simulink model "AirTableModel"  (R2021a)
settings: Solver=FixedStepAuto  StartTime=0.0  StopTime=endTime  FixedStep=dynamicsRate  RelTol=1e-3  EnableMultiTasking=on
InitFcn:
  | loadThrusterData
  | loadSensorData
values from neighbouring files (symbols this model uses):
  AccelIIR_Den = [1.000000000000000  -1.561018075800718   0.641351538057563]    [loadSensorData.m]
  AccelIIR_Num = [0.020083365564211   0.040166731128423   0.020083365564211]    [loadSensorData.m]
  cameraVec = [1 0 0]    [loadSensorData.m]
  controlRate = 0.025    [loadBusData.m]
  controlType = 1    [loadBusData.m]    (also in loadControlData.m = 2)
  dynamicsRate = 0.005    [loadBusData.m]
  finalRangeAttitude = [0 0 90]*dtr    [loadGuidanceData.m]
  finalRangeValue = 0.25    [loadGuidanceData.m]
  initialCovariance = diag([999999 999999 999999 999999 999999 999999])    [loadSensorData.m]
  initialNavState = [initialState + [0.01 -0.01 1e-3 0 0 1e-3]]    [loadSensorData.m]
  Kd = [x(4) x(5) 0 0 0 x(6)]    [executeSim.m]    (also in loadBusData.m = [500.0000  501.0938 0 0 0 18.4778]; loadControlData.m = [80 80 0 0 0 5] .*[.2 .2  0 0 0 .1]; planarPIDControl.m = [kd(1) 0 0; 0 kd(2) 0; 0 0 kd(3)])
  Ki = [x(7) x(8) 0 0 0 x(9)]    [executeSim.m]    (also in loadBusData.m = [1.0000    1.0313   0 0 0 58.1181]; loadControlData.m = [4  4  0 0 0 1] .*[1   1  0 0 0 .5]; planarPIDControl.m = [ki(1) 0 0; 0 ki(2) 0; 0 0 ki(3)])
  Kp = [x(1) x(2) 0 0 0 x(3)]    [executeSim.m]    (also in loadBusData.m = [500.0000  246.1321 0 0 0 50.1701]; loadControlData.m = [70 70 0 0 0 20].*[.2 .2  0 0 0 .25]; planarPIDControl.m = [kp(1) 0 0; 0 kp(2) 0; 0 0 kp(3)])
  M_Tracker_To_Body = [1 0 0; 0 1 0; 0 0 1]    [loadSensorData.m]
  measurementNoise = [1 .0873 0.0017 2].* [.01 1 1 .01]    [loadSensorData.m]
  processNoise = 0    [loadSensorData.m]
  R_Tracker_To_ECEF = [0 0 0]    [loadSensorData.m]
  rangeSensorAngBody = [0; 90*dtr; 180*dtr; 270*dtr]    [loadSensorData.m]
  rangeSensorFOV = [0*dtr; 0*dtr; 0*dtr; 0*dtr]    [loadSensorData.m]
  rangeSensorIdx = 1    [loadGuidanceData.m]
  SMGains = x    [executeSim.m]    (also in loadBusData.m = [2.0801    3.0489    8.9333    4.9881    3.0029    9.5293   ; loadControlData.m = [3.5078    3.9888    6.3119    1.8214    4.7749    7.3059   )
  useRangeGuid = 0    [loadGuidanceData.m]
  VelIIR_Den = [1.000000000000000  -1.944477657767094   0.945977936232282]    [loadSensorData.m]
  VelIIR_Num = [0.375069616296964   0.750139232593927   0.375069616296964]*1e-3    [loadSensorData.m]
  wallBounds = [wallA; wallB; wallC; wallD]    [loadSensorData.m]
undefined symbols (not defined in the file or in its folder): initialState, navType, PPGains, rangeSensorLocBody, refIdx, targetVec
libraries: simulink x25
(part 2 of 2)

== system AirTableModel/Executive/Guidance/RangeSensorGuidance ==
  In1 : Inport
  rangeSensorData : Inport  Port=2
  Bus Selector2 : BusSelector  OutputSignals=TranState_ECEF.R_Sys_ECEF,RotState_Body_ECEF.ECEF_To_Body_Euler,TranState_ECEF.V_Sys_ECEF,RotState_Body_ECEF.BodyRates_wrt_ECEF_In_Body
  Mux3 : Mux
  RangeGuidance : ModelReference  ModelNameDialog=RangeGuidance  SimulationMode=Normal  ModelReferenceVersion=6.8
      settings: PortSchema="{\"entries\":[{\"content\":{\"sides\":[{\"content\":{\"connectorIds\":[\"In1\",\"In2\",\"In4\",\"In3\",\"In6\",\"In5\"]},\"type\":\"ConnectorPlacement.EquallySpacedRectSide\",\"uuid\":\"ce2fad76-9ac2-4efb-9069-bf35fa3b239d\"},{\"content\":{\"connectorIds\":[\"Out1\",\"Out2\",\"Out3\",\"Out4\",\"Out5\"],\"side\":\"RIGHT\"},\"type\":\"ConnectorPlacement.EquallySpacedRectSide\",\"uuid\":\"aa89394c-f584-49d8-8867-538537a392b4\"},{\"content\":{\"connectorIds\":[],\"side\":\"TOP\"},\"type\":\"ConnectorPlacement.EquallySpacedRectSide\",\"uuid\":\"b335fb80-6985-455b-ae93-e5936637ca43\"}]},\"type\":\"ConnectorPlacement.EquallySpacedConnector\",\"uuid\":\"e071ca64-4f20-42cf-9888-09e4aeb0f4d6\"}],\"packageUris\":[\"http://schema.mathworks.com/mf0/Connector/R2020b\"],\"version\":\"1.0\"}"
  To Workspace4 : ToWorkspace  VariableName=sensorBodyVec1  SaveFormat=Timeseries  SampleTime=-1
  To Workspace5 : ToWorkspace  VariableName=rangeError1  SaveFormat=Timeseries  SampleTime=-1
  To Workspace6 : ToWorkspace  VariableName=rangeErrorECEF1  SaveFormat=Timeseries  SampleTime=-1
  To Workspace7 : ToWorkspace  VariableName=desiredPosECEF1  SaveFormat=Timeseries  SampleTime=-1
  To Workspace8 : ToWorkspace  VariableName=sensorECEFVec1  SaveFormat=Timeseries  SampleTime=-1
  rangeAttitude : Constant  Value=finalRangeAttitude
  rangeSensorAngle : Constant  Value=rangeSensorAngBody
  rangeSensorIdx : Constant  Value=rangeSensorIdx
  rangeValue : Constant  Value=finalRangeValue
  desiredPosECEF : Outport
  wires:
  In1/1 -> Bus Selector2/1
  Bus Selector2/3 -> Mux3/3  "<V_Sys_ECEF>"
  RangeGuidance/3 -> To Workspace5/1
  Mux3/1 -> RangeGuidance/1
  rangeAttitude/1 -> RangeGuidance/2
  Bus Selector2/4 -> Mux3/4  "<BodyRates_wrt_ECEF_In_Body>"
  Bus Selector2/2 -> Mux3/2  "<ECEF_To_Body_Euler>"
  RangeGuidance/2 -> To Workspace4/1
  rangeSensorData/1 -> RangeGuidance/4
  RangeGuidance/4 -> To Workspace6/1
  Bus Selector2/1 -> Mux3/1  "<R_Sys_ECEF>"
  RangeGuidance/1 -> desiredPosECEF/1, To Workspace7/1
  RangeGuidance/5 -> To Workspace8/1
  rangeSensorIdx/1 -> RangeGuidance/3
  rangeSensorAngle/1 -> RangeGuidance/5
  rangeValue/1 -> RangeGuidance/6

== system AirTableModel/Executive/Guidance/ReferenceTrajectoryGuidance ==
  Time : Inport
  refTraj : Inport  Port=2
  controlType : Inport  Port=3
  If : If  IfExpression=u1 == 3
  LookupRefTrajInterpolate : Subsystem  TreatAsAtomicUnit=on
  LookupRefTrajNoInterp : Subsystem  TreatAsAtomicUnit=on
  Merge : Merge
  referenceValues : Outport
  wires:
  refTraj/1 -> LookupRefTrajInterpolate/2(refTraj), LookupRefTrajNoInterp/2(refTraj)
  Merge/1 -> referenceValues/1
  controlType/1 -> If/1
  If/1 -> LookupRefTrajNoInterp/Action
  If/2 -> LookupRefTrajInterpolate/Action
  LookupRefTrajNoInterp/1(referenceValues) -> Merge/1
  LookupRefTrajInterpolate/1(referenceValues) -> Merge/2
  Time/1 -> LookupRefTrajInterpolate/1(Time), LookupRefTrajNoInterp/1(Time)

== system AirTableModel/Navigation/FilterSensorData/FilterVector ==
  Signal : Inport
  Numerator : Inport  Port=2
  Denominator : Inport  Port=3
  IC : Inport  Port=4
  Discrete Filter : DiscreteFilter  NumeratorSource=Input port  DenominatorSource=Input port  InitialStatesSource=Input port  a0EqualsOne=on
      settings: InputPortMap=u0,p1,p3,p5
  Discrete Filter1 : DiscreteFilter  NumeratorSource=Input port  DenominatorSource=Input port  InitialStatesSource=Input port  a0EqualsOne=on
      settings: InputPortMap=u0,p1,p3,p5
  Discrete Filter2 : DiscreteFilter  NumeratorSource=Input port  DenominatorSource=Input port  InitialStatesSource=Input port  a0EqualsOne=on
      settings: InputPortMap=u0,p1,p3,p5
  Mux1 : Mux  Inputs=3
  X : Selector  InputPortWidth=3  IndexOptions=Index vector (dialog)  Indices=1  OutputSizes=1
  X3 : Selector  InputPortWidth=3  IndexOptions=Index vector (dialog)  Indices=1  OutputSizes=1
  Y : Selector  InputPortWidth=3  IndexOptions=Index vector (dialog)  Indices=2  OutputSizes=1
  Y3 : Selector  InputPortWidth=3  IndexOptions=Index vector (dialog)  Indices=2  OutputSizes=1
  Z : Selector  InputPortWidth=3  IndexOptions=Index vector (dialog)  Indices=3  OutputSizes=1
  Z3 : Selector  InputPortWidth=3  IndexOptions=Index vector (dialog)  Indices=3  OutputSizes=1
  Out1 : Outport
  wires:
  Signal/1 -> Z/1, Y/1, X/1
  IC/1 -> Z3/1, X3/1, Y3/1
  Mux1/1 -> Out1/1
  Discrete Filter/1 -> Mux1/1
  X/1 -> Discrete Filter/1
  X3/1 -> Discrete Filter/4
  Y/1 -> Discrete Filter1/1
  Y3/1 -> Discrete Filter1/4
  Z/1 -> Discrete Filter2/1
  Z3/1 -> Discrete Filter2/4
  Discrete Filter1/1 -> Mux1/2
  Discrete Filter2/1 -> Mux1/3
  Numerator/1 -> Discrete Filter1/2, Discrete Filter/2, Discrete Filter2/2
  Denominator/1 -> Discrete Filter2/3, Discrete Filter1/3, Discrete Filter/3

== system AirTableModel/Navigation/FilterSensorData/FilterVector1 ==
  Signal : Inport
  Numerator : Inport  Port=2
  Denominator : Inport  Port=3
  IC : Inport  Port=4
  Discrete Filter : DiscreteFilter  NumeratorSource=Input port  DenominatorSource=Input port  InitialStatesSource=Input port  a0EqualsOne=on
      settings: InputPortMap=u0,p1,p3,p5
  Discrete Filter1 : DiscreteFilter  NumeratorSource=Input port  DenominatorSource=Input port  InitialStatesSource=Input port  a0EqualsOne=on
      settings: InputPortMap=u0,p1,p3,p5
  Discrete Filter2 : DiscreteFilter  NumeratorSource=Input port  DenominatorSource=Input port  InitialStatesSource=Input port  a0EqualsOne=on
      settings: InputPortMap=u0,p1,p3,p5
  Mux1 : Mux  Inputs=3
  X : Selector  InputPortWidth=3  IndexOptions=Index vector (dialog)  Indices=1  OutputSizes=1
  X3 : Selector  InputPortWidth=3  IndexOptions=Index vector (dialog)  Indices=1  OutputSizes=1
  Y : Selector  InputPortWidth=3  IndexOptions=Index vector (dialog)  Indices=2  OutputSizes=1
  Y3 : Selector  InputPortWidth=3  IndexOptions=Index vector (dialog)  Indices=2  OutputSizes=1
  Z : Selector  InputPortWidth=3  IndexOptions=Index vector (dialog)  Indices=3  OutputSizes=1
  Z3 : Selector  InputPortWidth=3  IndexOptions=Index vector (dialog)  Indices=3  OutputSizes=1
  Out1 : Outport
  wires:
  Signal/1 -> Z/1, Y/1, X/1
  IC/1 -> Z3/1, X3/1, Y3/1
  Mux1/1 -> Out1/1
  Discrete Filter/1 -> Mux1/1
  X/1 -> Discrete Filter/1
  X3/1 -> Discrete Filter/4
  Y/1 -> Discrete Filter1/1
  Y3/1 -> Discrete Filter1/4
  Z/1 -> Discrete Filter2/1
  Z3/1 -> Discrete Filter2/4
  Discrete Filter1/1 -> Mux1/2
  Discrete Filter2/1 -> Mux1/3
  Numerator/1 -> Discrete Filter1/2, Discrete Filter/2, Discrete Filter2/2
  Denominator/1 -> Discrete Filter2/3, Discrete Filter1/3, Discrete Filter/3

== system AirTableModel/Navigation/FilterSensorData/FilterVector2 ==
  Signal : Inport
  Numerator : Inport  Port=2
  Denominator : Inport  Port=3
  IC : Inport  Port=4
  Discrete Filter : DiscreteFilter  NumeratorSource=Input port  DenominatorSource=Input port  InitialStatesSource=Input port  a0EqualsOne=on
      settings: InputPortMap=u0,p1,p3,p5
  Discrete Filter1 : DiscreteFilter  NumeratorSource=Input port  DenominatorSource=Input port  InitialStatesSource=Input port  a0EqualsOne=on
      settings: InputPortMap=u0,p1,p3,p5
  Discrete Filter2 : DiscreteFilter  NumeratorSource=Input port  DenominatorSource=Input port  InitialStatesSource=Input port  a0EqualsOne=on
      settings: InputPortMap=u0,p1,p3,p5
  Mux1 : Mux  Inputs=3
  X : Selector  InputPortWidth=3  IndexOptions=Index vector (dialog)  Indices=1  OutputSizes=1
  X3 : Selector  InputPortWidth=3  IndexOptions=Index vector (dialog)  Indices=1  OutputSizes=1
  Y : Selector  InputPortWidth=3  IndexOptions=Index vector (dialog)  Indices=2  OutputSizes=1
  Y3 : Selector  InputPortWidth=3  IndexOptions=Index vector (dialog)  Indices=2  OutputSizes=1
  Z : Selector  InputPortWidth=3  IndexOptions=Index vector (dialog)  Indices=3  OutputSizes=1
  Z3 : Selector  InputPortWidth=3  IndexOptions=Index vector (dialog)  Indices=3  OutputSizes=1
  Out1 : Outport
  wires:
  Signal/1 -> Z/1, Y/1, X/1
  IC/1 -> Z3/1, X3/1, Y3/1
  Mux1/1 -> Out1/1
  Discrete Filter/1 -> Mux1/1
  X/1 -> Discrete Filter/1
  X3/1 -> Discrete Filter/4
  Y/1 -> Discrete Filter1/1
  Y3/1 -> Discrete Filter1/4
  Z/1 -> Discrete Filter2/1
  Z3/1 -> Discrete Filter2/4
  Discrete Filter1/1 -> Mux1/2
  Discrete Filter2/1 -> Mux1/3
  Numerator/1 -> Discrete Filter1/2, Discrete Filter/2, Discrete Filter2/2
  Denominator/1 -> Discrete Filter2/3, Discrete Filter1/3, Discrete Filter/3

== system AirTableModel/Navigation/FilterSensorData/FilterVector3 ==
  Signal : Inport
  Numerator : Inport  Port=2
  Denominator : Inport  Port=3
  IC : Inport  Port=4
  Discrete Filter : DiscreteFilter  NumeratorSource=Input port  DenominatorSource=Input port  InitialStatesSource=Input port  a0EqualsOne=on
      settings: InputPortMap=u0,p1,p3,p5
  Discrete Filter1 : DiscreteFilter  NumeratorSource=Input port  DenominatorSource=Input port  InitialStatesSource=Input port  a0EqualsOne=on
      settings: InputPortMap=u0,p1,p3,p5
  Discrete Filter2 : DiscreteFilter  NumeratorSource=Input port  DenominatorSource=Input port  InitialStatesSource=Input port  a0EqualsOne=on
      settings: InputPortMap=u0,p1,p3,p5
  Mux1 : Mux  Inputs=3
  X : Selector  InputPortWidth=3  IndexOptions=Index vector (dialog)  Indices=1  OutputSizes=1
  X3 : Selector  InputPortWidth=3  IndexOptions=Index vector (dialog)  Indices=1  OutputSizes=1
  Y : Selector  InputPortWidth=3  IndexOptions=Index vector (dialog)  Indices=2  OutputSizes=1
  Y3 : Selector  InputPortWidth=3  IndexOptions=Index vector (dialog)  Indices=2  OutputSizes=1
  Z : Selector  InputPortWidth=3  IndexOptions=Index vector (dialog)  Indices=3  OutputSizes=1
  Z3 : Selector  InputPortWidth=3  IndexOptions=Index vector (dialog)  Indices=3  OutputSizes=1
  Out1 : Outport
  wires:
  Signal/1 -> Z/1, Y/1, X/1
  IC/1 -> Z3/1, X3/1, Y3/1
  Mux1/1 -> Out1/1
  Discrete Filter/1 -> Mux1/1
  X/1 -> Discrete Filter/1
  X3/1 -> Discrete Filter/4
  Y/1 -> Discrete Filter1/1
  Y3/1 -> Discrete Filter1/4
  Z/1 -> Discrete Filter2/1
  Z3/1 -> Discrete Filter2/4
  Discrete Filter1/1 -> Mux1/2
  Discrete Filter2/1 -> Mux1/3
  Numerator/1 -> Discrete Filter1/2, Discrete Filter/2, Discrete Filter2/2
  Denominator/1 -> Discrete Filter2/3, Discrete Filter1/3, Discrete Filter/3

== system AirTableModel/Navigation/FilterSensorData/FilterVector4 ==
  Signal : Inport
  Numerator : Inport  Port=2
  Denominator : Inport  Port=3
  IC : Inport  Port=4
  Discrete Filter : DiscreteFilter  NumeratorSource=Input port  DenominatorSource=Input port  InitialStatesSource=Input port  a0EqualsOne=on
      settings: InputPortMap=u0,p1,p3,p5
  Discrete Filter1 : DiscreteFilter  NumeratorSource=Input port  DenominatorSource=Input port  InitialStatesSource=Input port  a0EqualsOne=on
      settings: InputPortMap=u0,p1,p3,p5
  Discrete Filter2 : DiscreteFilter  NumeratorSource=Input port  DenominatorSource=Input port  InitialStatesSource=Input port  a0EqualsOne=on
      settings: InputPortMap=u0,p1,p3,p5
  Mux1 : Mux  Inputs=3
  X : Selector  InputPortWidth=3  IndexOptions=Index vector (dialog)  Indices=1  OutputSizes=1
  X3 : Selector  InputPortWidth=3  IndexOptions=Index vector (dialog)  Indices=1  OutputSizes=1
  Y : Selector  InputPortWidth=3  IndexOptions=Index vector (dialog)  Indices=2  OutputSizes=1
  Y3 : Selector  InputPortWidth=3  IndexOptions=Index vector (dialog)  Indices=2  OutputSizes=1
  Z : Selector  InputPortWidth=3  IndexOptions=Index vector (dialog)  Indices=3  OutputSizes=1
  Z3 : Selector  InputPortWidth=3  IndexOptions=Index vector (dialog)  Indices=3  OutputSizes=1
  Out1 : Outport
  wires:
  Signal/1 -> Z/1, Y/1, X/1
  IC/1 -> Z3/1, X3/1, Y3/1
  Mux1/1 -> Out1/1
  Discrete Filter/1 -> Mux1/1
  X/1 -> Discrete Filter/1
  X3/1 -> Discrete Filter/4
  Y/1 -> Discrete Filter1/1
  Y3/1 -> Discrete Filter1/4
  Z/1 -> Discrete Filter2/1
  Z3/1 -> Discrete Filter2/4
  Discrete Filter1/1 -> Mux1/2
  Discrete Filter2/1 -> Mux1/3
  Numerator/1 -> Discrete Filter1/2, Discrete Filter/2, Discrete Filter2/2
  Denominator/1 -> Discrete Filter2/3, Discrete Filter1/3, Discrete Filter/3

== system AirTableModel/Process Inputs/Variant Subsystem/UseInputPorts ==
  refIdx : Inport
  navType : Inport  Port=2
  controlType : Inport  Port=3  OutDataTypeStr=uint8  PortDimensions=1
  refIdxOut : Outport
  navTypeOut : Outport  Port=2
  controlTypeOut : Outport  Port=3
  wires:
  refIdx/1 -> refIdxOut/1
  navType/1 -> navTypeOut/1
  controlType/1 -> controlTypeOut/1

== system AirTableModel/Process Inputs/Variant Subsystem/UseWorkspaceData ==
  controlType : Constant  Value=controlType
  navType : Constant  Value=navType
  refIdx : Constant  Value=refIdx
  refIdxOut : Outport
  navTypeOut : Outport  Port=2
  controlTypeOut : Outport  Port=3
  wires:
  refIdx/1 -> refIdxOut/1
  navType/1 -> navTypeOut/1
  controlType/1 -> controlTypeOut/1

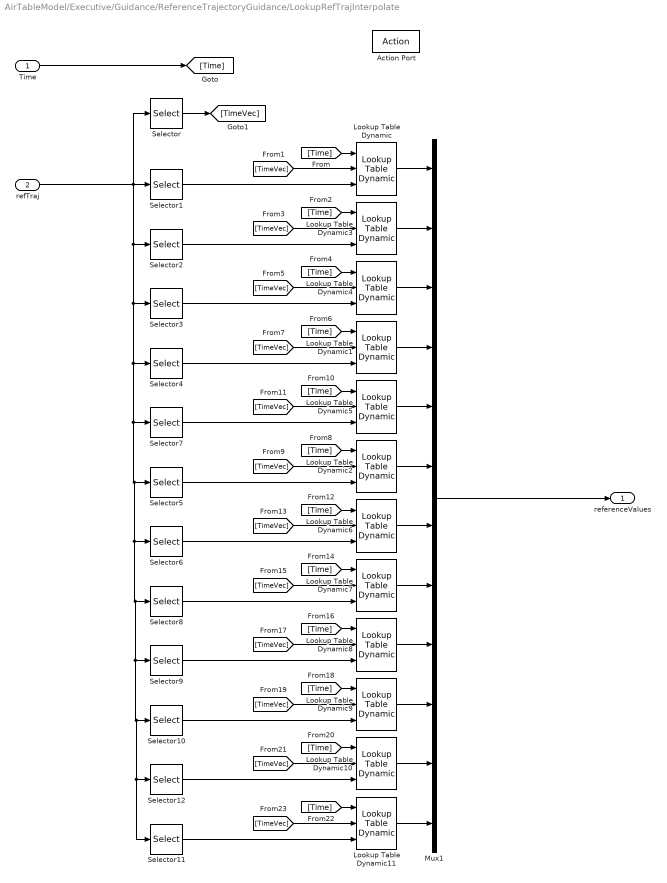
== system AirTableModel/Executive/Guidance/ReferenceTrajectoryGuidance/LookupRefTrajInterpolate ==
  Time : Inport
  refTraj : Inport  Port=2
  Action Port : ActionPort  ActionPortLabel=else
  Lookup Table Dynamic{,1..11} (12 alike) : simulink/Lookup Tables/Lookup Table Dynamic  LookUpMeth=Interpolation-Use End Values  OutDataType=fixdt('double')  OutScaling=[]  OutputDataTypeScalingMode=Specify via dialog  OutDataTypeStr=double  DoSatur=off
  Mux1 : Mux  Inputs=12
  Selector : Selector  NumberOfDimensions=2  InputPortWidth=3  IndexOptions=Select all,Index vector (dialog)  Indices=1,1  OutputSizes=1,1
  Selector1 : Selector  NumberOfDimensions=2  InputPortWidth=3  IndexOptions=Select all,Index vector (dialog)  Indices=1,2  OutputSizes=1,1
  Selector10 : Selector  NumberOfDimensions=2  InputPortWidth=3  IndexOptions=Select all,Index vector (dialog)  Indices=1,11  OutputSizes=1,1
  Selector11 : Selector  NumberOfDimensions=2  InputPortWidth=3  IndexOptions=Select all,Index vector (dialog)  Indices=1,13  OutputSizes=1,1
  Selector12 : Selector  NumberOfDimensions=2  InputPortWidth=3  IndexOptions=Select all,Index vector (dialog)  Indices=1,12  OutputSizes=1,1
  Selector2 : Selector  NumberOfDimensions=2  InputPortWidth=3  IndexOptions=Select all,Index vector (dialog)  Indices=1,3  OutputSizes=1,1
  Selector3 : Selector  NumberOfDimensions=2  InputPortWidth=3  IndexOptions=Select all,Index vector (dialog)  Indices=1,4  OutputSizes=1,1
  Selector4 : Selector  NumberOfDimensions=2  InputPortWidth=3  IndexOptions=Select all,Index vector (dialog)  Indices=1,5  OutputSizes=1,1
  Selector5 : Selector  NumberOfDimensions=2  InputPortWidth=3  IndexOptions=Select all,Index vector (dialog)  Indices=1,7  OutputSizes=1,1
  Selector6 : Selector  NumberOfDimensions=2  InputPortWidth=3  IndexOptions=Select all,Index vector (dialog)  Indices=1,8  OutputSizes=1,1
  Selector7 : Selector  NumberOfDimensions=2  InputPortWidth=3  IndexOptions=Select all,Index vector (dialog)  Indices=1,6  OutputSizes=1,1
  Selector8 : Selector  NumberOfDimensions=2  InputPortWidth=3  IndexOptions=Select all,Index vector (dialog)  Indices=1,9  OutputSizes=1,1
  Selector9 : Selector  NumberOfDimensions=2  InputPortWidth=3  IndexOptions=Select all,Index vector (dialog)  Indices=1,10  OutputSizes=1,1
  referenceValues : Outport  VectorParamsAs1DForOutWhenUnconnected=off
  wires:
  Selector9/1 -> Lookup Table Dynamic8/3
  [TimeVec] -> Lookup Table Dynamic8/2
  Selector8/1 -> Lookup Table Dynamic7/3
  [TimeVec] -> Lookup Table Dynamic4/2
  [Time] -> Lookup Table Dynamic2/1
  [Time] -> Lookup Table Dynamic1/1
  Selector7/1 -> Lookup Table Dynamic5/3
  [Time] -> Lookup Table Dynamic4/1
  [TimeVec] -> Lookup Table Dynamic7/2
  [TimeVec] -> Lookup Table Dynamic/2
  Lookup Table Dynamic/1 -> Mux1/1
  Lookup Table Dynamic3/1 -> Mux1/2
  [Time] -> Lookup Table Dynamic/1
  Selector5/1 -> Lookup Table Dynamic2/3
  [TimeVec] -> Lookup Table Dynamic5/2
  Mux1/1 -> referenceValues/1
  Selector/1 -> [TimeVec]
  [TimeVec] -> Lookup Table Dynamic3/2
  [Time] -> Lookup Table Dynamic6/1
  [Time] -> Lookup Table Dynamic9/1
  Lookup Table Dynamic7/1 -> Mux1/8
  Lookup Table Dynamic4/1 -> Mux1/3
  Lookup Table Dynamic9/1 -> Mux1/10
  Lookup Table Dynamic10/1 -> Mux1/11
  Selector4/1 -> Lookup Table Dynamic1/3
  Selector1/1 -> Lookup Table Dynamic/3
  Selector2/1 -> Lookup Table Dynamic3/3
  Selector6/1 -> Lookup Table Dynamic6/3
  [TimeVec] -> Lookup Table Dynamic6/2
  Lookup Table Dynamic11/1 -> Mux1/12
  [TimeVec] -> Lookup Table Dynamic10/2
  Lookup Table Dynamic5/1 -> Mux1/5
  [Time] -> Lookup Table Dynamic3/1
  Selector10/1 -> Lookup Table Dynamic9/3
  [Time] -> Lookup Table Dynamic11/1
  [Time] -> Lookup Table Dynamic10/1
  Lookup Table Dynamic1/1 -> Mux1/4
  [TimeVec] -> Lookup Table Dynamic1/2
  [TimeVec] -> Lookup Table Dynamic9/2
  [TimeVec] -> Lookup Table Dynamic2/2
  refTraj/1 -> Selector1/1, Selector/1, Selector2/1, Selector3/1, Selector4/1, Selector7/1, Selector11/1, Selector12/1, Selector10/1, Selector9/1, Selector8/1, Selector6/1, Selector5/1
  [Time] -> Lookup Table Dynamic8/1
  Lookup Table Dynamic6/1 -> Mux1/7
  Lookup Table Dynamic2/1 -> Mux1/6
  Selector3/1 -> Lookup Table Dynamic4/3
  Selector11/1 -> Lookup Table Dynamic11/3
  [Time] -> Lookup Table Dynamic5/1
  Selector12/1 -> Lookup Table Dynamic10/3
  Lookup Table Dynamic8/1 -> Mux1/9
  Time/1 -> [Time]
  [Time] -> Lookup Table Dynamic7/1
  [TimeVec] -> Lookup Table Dynamic11/2

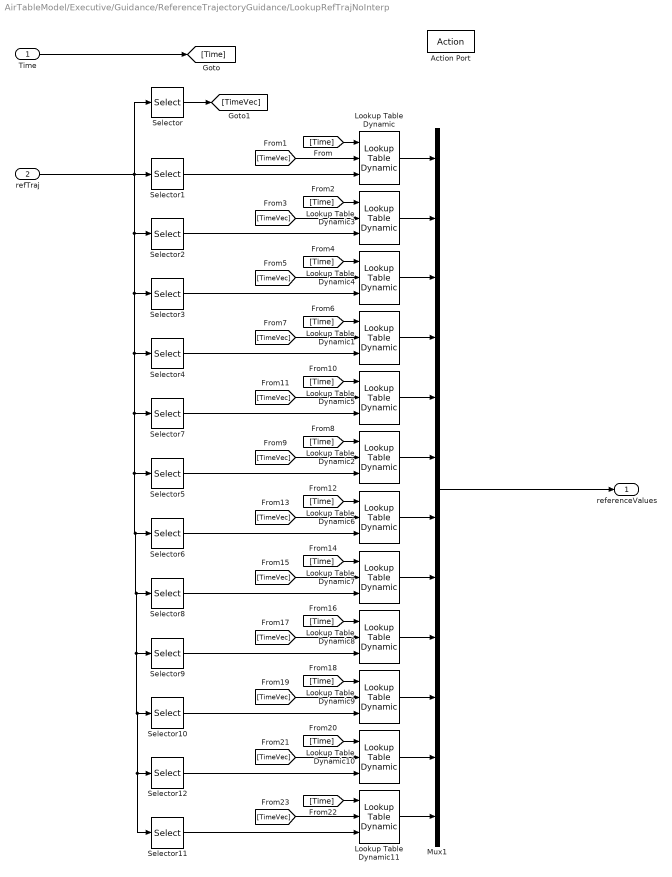
== system AirTableModel/Executive/Guidance/ReferenceTrajectoryGuidance/LookupRefTrajNoInterp ==
  Time : Inport
  refTraj : Inport  Port=2
  Action Port : ActionPort  ActionPortLabel=if(u1 == 3)
  Lookup Table Dynamic{,1..11} (12 alike) : simulink/Lookup Tables/Lookup Table Dynamic  LookUpMeth=Use Input Above  OutDataType=fixdt('double')  OutScaling=[]  OutputDataTypeScalingMode=Specify via dialog  OutDataTypeStr=double  DoSatur=off
  Mux1 : Mux  Inputs=12
  Selector : Selector  NumberOfDimensions=2  InputPortWidth=3  IndexOptions=Select all,Index vector (dialog)  Indices=1,1  OutputSizes=1,1
  Selector1 : Selector  NumberOfDimensions=2  InputPortWidth=3  IndexOptions=Select all,Index vector (dialog)  Indices=1,2  OutputSizes=1,1
  Selector10 : Selector  NumberOfDimensions=2  InputPortWidth=3  IndexOptions=Select all,Index vector (dialog)  Indices=1,11  OutputSizes=1,1
  Selector11 : Selector  NumberOfDimensions=2  InputPortWidth=3  IndexOptions=Select all,Index vector (dialog)  Indices=1,13  OutputSizes=1,1
  Selector12 : Selector  NumberOfDimensions=2  InputPortWidth=3  IndexOptions=Select all,Index vector (dialog)  Indices=1,12  OutputSizes=1,1
  Selector2 : Selector  NumberOfDimensions=2  InputPortWidth=3  IndexOptions=Select all,Index vector (dialog)  Indices=1,3  OutputSizes=1,1
  Selector3 : Selector  NumberOfDimensions=2  InputPortWidth=3  IndexOptions=Select all,Index vector (dialog)  Indices=1,4  OutputSizes=1,1
  Selector4 : Selector  NumberOfDimensions=2  InputPortWidth=3  IndexOptions=Select all,Index vector (dialog)  Indices=1,5  OutputSizes=1,1
  Selector5 : Selector  NumberOfDimensions=2  InputPortWidth=3  IndexOptions=Select all,Index vector (dialog)  Indices=1,7  OutputSizes=1,1
  Selector6 : Selector  NumberOfDimensions=2  InputPortWidth=3  IndexOptions=Select all,Index vector (dialog)  Indices=1,8  OutputSizes=1,1
  Selector7 : Selector  NumberOfDimensions=2  InputPortWidth=3  IndexOptions=Select all,Index vector (dialog)  Indices=1,6  OutputSizes=1,1
  Selector8 : Selector  NumberOfDimensions=2  InputPortWidth=3  IndexOptions=Select all,Index vector (dialog)  Indices=1,9  OutputSizes=1,1
  Selector9 : Selector  NumberOfDimensions=2  InputPortWidth=3  IndexOptions=Select all,Index vector (dialog)  Indices=1,10  OutputSizes=1,1
  referenceValues : Outport  VectorParamsAs1DForOutWhenUnconnected=off
  wires:
  Lookup Table Dynamic7/1 -> Mux1/8
  Lookup Table Dynamic8/1 -> Mux1/9
  [Time] -> Lookup Table Dynamic8/1
  [TimeVec] -> Lookup Table Dynamic8/2
  [TimeVec] -> Lookup Table Dynamic11/2
  [Time] -> Lookup Table Dynamic7/1
  Selector11/1 -> Lookup Table Dynamic11/3
  Lookup Table Dynamic6/1 -> Mux1/7
  Selector9/1 -> Lookup Table Dynamic8/3
  Lookup Table Dynamic9/1 -> Mux1/10
  Selector4/1 -> Lookup Table Dynamic1/3
  Selector1/1 -> Lookup Table Dynamic/3
  [Time] -> Lookup Table Dynamic9/1
  [Time] -> Lookup Table Dynamic11/1
  Lookup Table Dynamic10/1 -> Mux1/11
  [TimeVec] -> Lookup Table Dynamic/2
  [TimeVec] -> Lookup Table Dynamic9/2
  Selector12/1 -> Lookup Table Dynamic10/3
  [TimeVec] -> Lookup Table Dynamic10/2
  Lookup Table Dynamic1/1 -> Mux1/4
  [TimeVec] -> Lookup Table Dynamic7/2
  Selector/1 -> [TimeVec]
  Selector8/1 -> Lookup Table Dynamic7/3
  [Time] -> Lookup Table Dynamic6/1
  [TimeVec] -> Lookup Table Dynamic2/2
  refTraj/1 -> Selector1/1, Selector/1, Selector2/1, Selector3/1, Selector4/1, Selector7/1, Selector11/1, Selector12/1, Selector10/1, Selector9/1, Selector8/1, Selector6/1, Selector5/1
  Selector6/1 -> Lookup Table Dynamic6/3
  [Time] -> Lookup Table Dynamic5/1
  Selector10/1 -> Lookup Table Dynamic9/3
  Lookup Table Dynamic11/1 -> Mux1/12
  [TimeVec] -> Lookup Table Dynamic1/2
  [TimeVec] -> Lookup Table Dynamic6/2
  Mux1/1 -> referenceValues/1
  [Time] -> Lookup Table Dynamic1/1
  Selector2/1 -> Lookup Table Dynamic3/3
  [Time] -> Lookup Table Dynamic10/1
  Selector5/1 -> Lookup Table Dynamic2/3
  [TimeVec] -> Lookup Table Dynamic3/2
  [Time] -> Lookup Table Dynamic3/1
  Selector3/1 -> Lookup Table Dynamic4/3
  Lookup Table Dynamic/1 -> Mux1/1
  Lookup Table Dynamic3/1 -> Mux1/2
  [TimeVec] -> Lookup Table Dynamic4/2
  [Time] -> Lookup Table Dynamic2/1
  Selector7/1 -> Lookup Table Dynamic5/3
  Lookup Table Dynamic4/1 -> Mux1/3
  Time/1 -> [Time]
  [TimeVec] -> Lookup Table Dynamic5/2
  Lookup Table Dynamic2/1 -> Mux1/6
  Lookup Table Dynamic5/1 -> Mux1/5
  [Time] -> Lookup Table Dynamic/1
  [Time] -> Lookup Table Dynamic4/1

== matlab function AirTableModel/Dynamics/Rotate_Vector ==
  data: vIn input; vOut output; quat input
function vOut  = fcn(vIn,quat)

quatT = quatconj(quat');
vOut = quatrotate(vIn,quatT)';

== matlab function AirTableModel/Navigation/EstimateStates/Rotate_Vector ==
  data: vIn input; vOut output; quat input
function vOut  = fcn(vIn,quat)

quatT = quatconj(quat');
vOut = quatrotate(vIn,quatT)';

== matlab function AirTableModel/Navigation/MATLAB Function1 ==
  data: thetaAng input; estAng output; targetVec input; cameraVec input
function estAng  = callestimateAttitude(thetaAng,targetVec,cameraVec)

[estAng] = estimateAttitude(thetaAng,targetVec,cameraVec);

== matlab function AirTableModel/Process Inputs/Create Reference Trajectory/MATLAB Function1 ==
  data: refIdx input; refTraj output; ICState input; controlType input; PositionData input; rawPosition input; RotationData input
function refTraj   = callreferenceTrajectory(refIdx,ICState,controlType,PositionData,rawPosition,RotationData)

[refTraj] = referenceTrajectory(ICState,refIdx,controlType,PositionData,rawPosition,RotationData);

== matlab function AirTableModel/Compute_Outputs/Rotate_Vector ==
  data: vIn input; vOut output; quat input
function vOut  = fcn(vIn,quat)

quatT = quatconj(quat');
vOut = quatrotate(vIn,quat')';

== matlab function AirTableModel/Process Inputs/MATLAB Function ==
  data: m output; Izz output
function [m,Izz] = callplanarMassProperties

[m, Izz] = planarMassProperties();

== matlab function AirTableModel/Process Inputs/IC_State/Form_ECEF_To_Body ==
  data: euler input; q output
function q  = fcn(euler)

q = EulerToquat_321(euler);

== matlab function AirTableModel/Compute_Outputs/Rotate_Vector1 ==
  data: vIn input; vOut output; quat input
function vOut  = fcn(vIn,quat)

quatT = quatconj(quat');
vOut = quatrotate(vIn,quat')';

== matlab function AirTableModel/Process Inputs/IC_State/Form_Body_Vec ==
  data: posECEF input; velECEF input; posBody output; velBody output; qin input
function [posBody,velBody] = fcn(posECEF,velECEF,qin)

posBody = quatrotate(posECEF,qin);
velBody = quatrotate(velECEF,qin);

== matlab function AirTableModel/Compute_Outputs/computeRangeData/MATLAB Function1 ==
  data: t input; range output; state input; rangeSensorLocBody input; rangeSensorAngBody input; rangeSensorFOV input; wallBounds input; rangeArray output
function [range,rangeArray] = callsenseWalls(t,state,rangeSensorLocBody,rangeSensorAngBody,rangeSensorFOV,wallBounds)

[range,rangeArray] = senseWalls(state,rangeSensorLocBody,rangeSensorAngBody,rangeSensorFOV,wallBounds);

== matlab function AirTableModel/Executive/MATLAB Function ==
  data: outGNCMode output; navState input; refTraj input; useRangeGuid input; inGNCMode input
function outGNCMode  = callgncExecutive(navState,refTraj,useRangeGuid,inGNCMode)

[outGNCMode] = gncExecutive(navState,refTraj,useRangeGuid,inGNCMode);

== matlab function AirTableModel/Navigation/EstimateStates/KalmanFilter ==
  data: t input; outputState output; inputState input; dt input; Pold input; measurements input; controlInputs input; massProperties input; pNoise input; mNoise input; Pnew output; K output
function [outputState,Pnew,K]  = callKalmanFilter(t,inputState,dt,Pold,measurements,controlInputs,massProperties,pNoise,mNoise)

[outputState,Pnew,K] = KalmanFilter(inputState,dt,Pold,measurements,controlInputs,massProperties,pNoise,mNoise);
